simulink model "export_archive_task"  (Simulink 3.00)
libraries: arclib x4, mathlib x4, analoglib x2, genlib x2

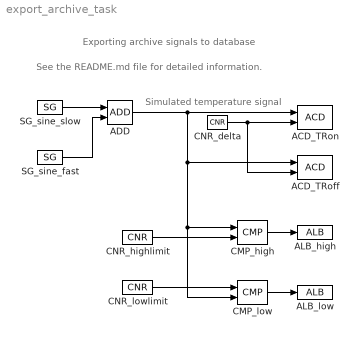
== system export_archive_task ==
  note: See the README.md file for detailed information.
  note: Exporting archive signals to database
  note: Simulated temperature signal
  ACD_TRoff : arclib/ACD  acls=8: Double  arc=1  id=2  tmin=0.1  tmax=5  TR=off  Desc=Simulated temperature signal, TR=off
  ACD_TRon : arclib/ACD  acls=8: Double  arc=1  id=1  tmin=0.1  tmax=5  TR=on  Desc=Simulated temperature signal, TR=on
  ADD : mathlib/ADD
  ALB_high : arclib/ALB  men=2: High-alarm enabled  arc=1  id=50  lvl=33  Desc=Value too high!
  ALB_low : arclib/ALB  men=2: High-alarm enabled  arc=1  id=51  lvl=32  Desc=Value too low!
  CMP_high : analoglib/CMP  hys=0.5
  CMP_low : analoglib/CMP  hys=0.5
  CNR_delta : mathlib/CNR  ycn=0.2
  CNR_highlimit : mathlib/CNR  ycn=11.0
  CNR_lowlimit : mathlib/CNR  ycn=-7.8
  SG_sine_fast : genlib/SG  isig=1: SINE  amp=3  freq=0.09  phase=0  ifrunit=1: Hz  iphunit=1: degrees
  SG_sine_slow : genlib/SG  isig=1: SINE  amp=10  freq=0.025  phase=0  ifrunit=1: Hz  iphunit=1: degrees
  wires:
  ADD/1 -> ACD_TRon/1, ACD_TRoff/1, CMP_high/1, CMP_low/2
  CMP_high/1 -> ALB_high/1
  CMP_low/1 -> ALB_low/1
  CNR_delta/1 -> ACD_TRoff/2, ACD_TRon/2
  CNR_highlimit/1 -> CMP_high/2
  CNR_lowlimit/1 -> CMP_low/1
  SG_sine_fast/1 -> ADD/2
  SG_sine_slow/1 -> ADD/1
